simulink model "ParameterAdaptive_control"  (R2013a)
settings: Solver=ode3  StartTime=0.0  StopTime=10.0  FixedStep=.01  RelTol=1e-3
values from neighbouring files (symbols this model uses):
  K = [Kp Kd]    [Hanoi_GUI.m]
  pihat0 = [Iz; m; mL; b]    [Hanoi_GUI.m]
undefined symbols (not defined in the file or in its folder): directhanoi, hanoidynamics, hanoitraj, inversehanoi, pihatdot, Y
settings Model: Creator=Sasha  LastModifiedBy=spaudel

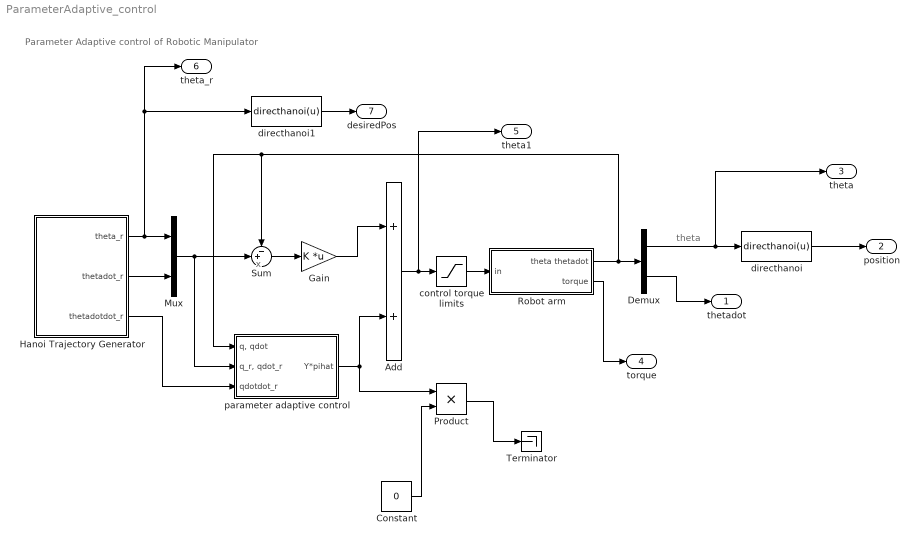
== system ParameterAdaptive_control ==
  note: Parameter Adaptive control of Robotic Manipulator
  note: x
  note: theta
  Add : Sum
  Constant : Constant  Value=0
  Demux : Demux  Outputs=2
  Gain : Gain  Gain=K  Multiplication=Matrix(K*u)
  Hanoi Trajectory Generator : Subsystem
  Mux : Mux  Inputs=2
  Product : Product
  Robot arm : Subsystem
  Sum : Sum  Inputs=-+|
  Terminator : Terminator
  control torque limits : Saturate  UpperLimit=3  LowerLimit=-3
  directhanoi : MATLABFcn  MATLABFcn=directhanoi(u)
  directhanoi1 : MATLABFcn  MATLABFcn=directhanoi(u)
  "parameter adaptive control " : Subsystem
  thetadot : Outport
  position : Outport  Port=2
  theta : Outport  Port=3
  torque : Outport  Port=4
  theta1 : Outport  Port=5
  theta_r : Outport  Port=6
  desiredPos : Outport  Port=7
  wires:
  Hanoi Trajectory Generator/2(thetadot_r) -> Mux/2
  Hanoi Trajectory Generator/1(theta_r) -> directhanoi1/1, theta_r/1, Mux/1
  Mux/1 -> "parameter adaptive control "/2("q_r, qdot_r"), Sum/2
  Sum/1 -> Gain/1
  Demux/2 -> thetadot/1
  directhanoi/1 -> position/1
  Robot arm/2(torque) -> torque/1
  Gain/1 -> Add/1
  Hanoi Trajectory Generator/3(thetadotdot_r) -> "parameter adaptive control "/3(qdotdot_r)
  "parameter adaptive control "/1(Y*pihat) -> Product/1, Add/2
  Demux/1 -> theta/1, directhanoi/1
  Add/1 -> theta1/1, control torque limits/1
  control torque limits/1 -> Robot arm/1(in)
  Robot arm/1(theta thetadot) -> Demux/1, "parameter adaptive control "/1("q, qdot"), Sum/1
  Constant/1 -> Product/2
  Product/1 -> Terminator/1
  directhanoi1/1 -> desiredPos/1

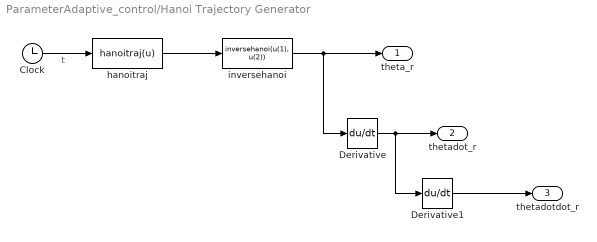
== system ParameterAdaptive_control/Hanoi Trajectory Generator ==
  note: t
  Clock : Clock
  Derivative : Derivative
  Derivative1 : Derivative
  hanoitraj : MATLABFcn  MATLABFcn=hanoitraj(u)
  inversehanoi : MATLABFcn  MATLABFcn=inversehanoi(u(1), u(2))
  theta_r : Outport
  thetadot_r : Outport  Port=2
  thetadotdot_r : Outport  Port=3
  wires:
  hanoitraj/1 -> inversehanoi/1
  Derivative/1 -> thetadot_r/1, Derivative1/1
  inversehanoi/1 -> theta_r/1, Derivative/1
  Clock/1 -> hanoitraj/1
  Derivative1/1 -> thetadotdot_r/1

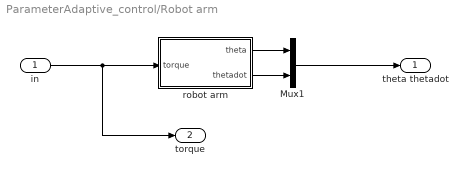
== system ParameterAdaptive_control/Robot arm ==
  in : Inport
  Mux1 : Mux  Inputs=2
  robot arm : Subsystem
  theta thetadot : Outport
  torque : Outport  Port=2
  wires:
  in/1 -> torque/1, robot arm/1(torque)
  robot arm/1(theta) -> Mux1/1
  robot arm/2(thetadot) -> Mux1/2
  Mux1/1 -> theta thetadot/1

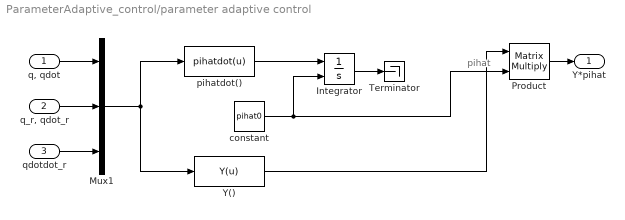
== system ParameterAdaptive_control/parameter adaptive control  ==
  note: pihat
  "q, qdot" : Inport
  "q_r, qdot_r" : Inport  Port=2
  qdotdot_r : Inport  Port=3
  Integrator : Integrator  InitialConditionSource=external
  Mux1 : Mux  Inputs=3
  Product : Product  Multiplication=Matrix(*)
  Terminator : Terminator
  Y() : MATLABFcn  MATLABFcn=Y(u)  Output1D=off
  constant : Constant  Value=pihat0
  pihatdot() : MATLABFcn  MATLABFcn=pihatdot(u)
  Y*pihat : Outport
  wires:
  "q, qdot"/1 -> Mux1/1
  qdotdot_r/1 -> Mux1/3
  "q_r, qdot_r"/1 -> Mux1/2
  pihatdot()/1 -> Integrator/1
  constant/1 -> Product/2, Integrator/2
  Mux1/1 -> Y()/1, pihatdot()/1
  Product/1 -> Y*pihat/1
  Y()/1 -> Product/1
  Integrator/1 -> Terminator/1

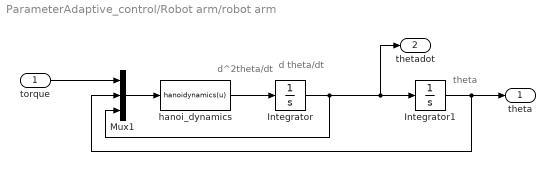
== system ParameterAdaptive_control/Robot arm/robot arm ==
  note: d^2theta/dt
  note: d theta/dt
  note: theta
  torque : Inport
  Integrator : Integrator  InitialCondition=[0;0]
  Integrator1 : Integrator  InitialCondition=[pi/2;-pi/2]
  Mux1 : Mux  Inputs=3
  hanoi_dynamics : MATLABFcn  MATLABFcn=hanoidynamics(u)
  theta : Outport
  thetadot : Outport  Port=2
  wires:
  hanoi_dynamics/1 -> Integrator/1
  Integrator/1 -> Mux1/3, thetadot/1, Integrator1/1
  Integrator1/1 -> theta/1, Mux1/2
  Mux1/1 -> hanoi_dynamics/1
  torque/1 -> Mux1/1
